simulink model "PID"  (R2023a)
settings: Solver=VariableStepDiscrete  StartTime=0.0  StopTime=10  RelTol=1e-3
values from neighbouring files (symbols this model uses):
  Kp = rand*15    [main.m]
  Td = rand*15    [main.m]
  Ti = rand*15    [main.m]
  Ts = rand*15    [main.m]
undefined symbols (not defined in the file or in its folder): DiscIntNeverNeededParam
settings Model: Creator=HW  LastModifiedBy=HW
settings SolverCC: ShapePreserveControl=EnableAll

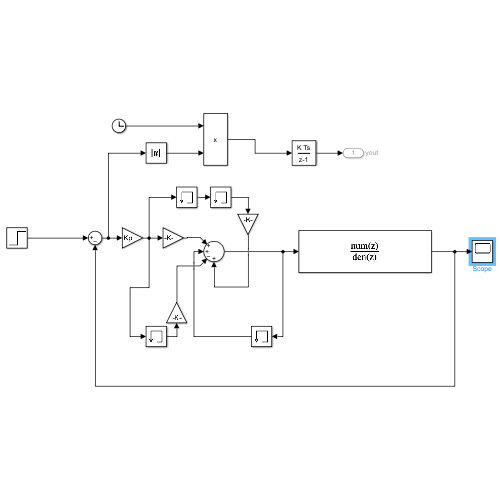
[thumbnail: Simulink's stored preview of the top-level diagram]
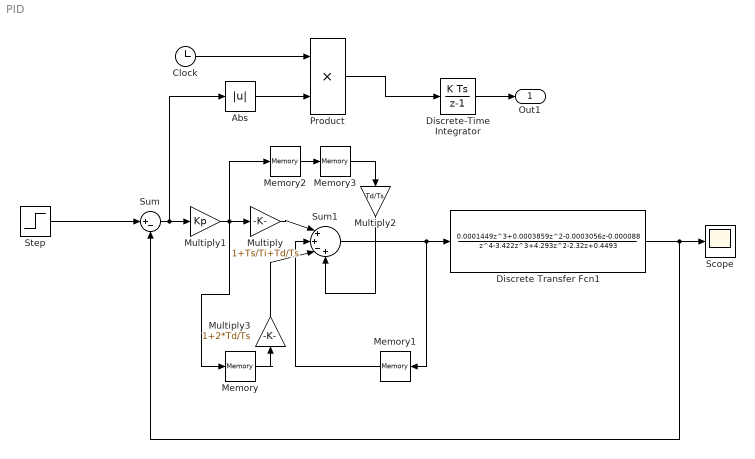
== system PID ==
  Abs : Abs  SaturateOnIntegerOverflow=off
  Clock : Clock
  Discrete Transfer Fcn1 : DiscreteTransferFcn  Numerator=[0.0001449 0.0003859 -0.0003056 -0.000088]  Denominator=[1 -3.422 4.293 -2.32 0.4493]  SampleTime=0.1
  Discrete-Time Integrator : DiscreteIntegrator  SampleTime=0.1  ICPrevOutput=DiscIntNeverNeededParam  ICPrevScaledInput=DiscIntNeverNeededParam
  Memory{,1..3} (4 alike) : Memory  InheritSampleTime=on
  Multiply : Gain  Gain=1+Ts/Ti+Td/Ts
  Multiply1 : Gain  Gain=Kp
  Multiply2 : Gain  Gain=Td/Ts
  Multiply3 : Gain  Gain=1+2*Td/Ts
  Product : Product
  Scope : Scope
  Step : Step  Time=0  SampleTime=0
  Sum : Sum  Inputs=|+-
  Sum1 : Sum  Inputs=|++-+
  Out1 : Outport  SignalName=yout
      settings: EnsureOutportIsVirtual=on
  wires:
  Discrete Transfer Fcn1/1 -> Scope/1, Sum/2
  Sum/1 -> Multiply1/1, Abs/1
  Clock/1 -> Product/1
  Abs/1 -> Product/2
  Product/1 -> Discrete-Time Integrator/1
  Step/1 -> Sum/1
  Multiply/1 -> Sum1/1
  Memory/1 -> Multiply3/1
  Sum1/1 -> Memory1/1, Discrete Transfer Fcn1/1
  Memory2/1 -> Memory3/1
  Memory3/1 -> Multiply2/1
  Multiply2/1 -> Sum1/4
  Multiply1/1 -> Memory2/1, Memory/1, Multiply/1
  Memory1/1 -> Sum1/2
  Multiply3/1 -> Sum1/3
  Discrete-Time Integrator/1 -> Out1/1
